simulink model "run_small_function_cov_bitadder"  (R2022b)
settings: Solver=VariableStepAuto  StartTime=0.0  StopTime=0.0  RelTol=1e-3
libraries: simulink x3193, hdlsllib x1590, ece1718_small_function x16
(part 4 of 26)

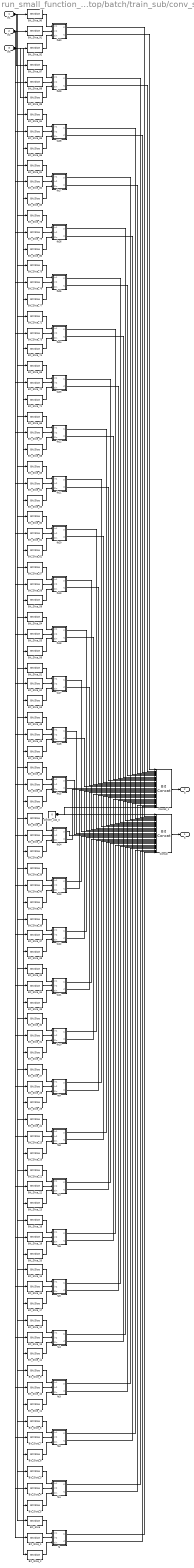
== system run_small_function_cov_bitadder/For Iterator Subsystem/train_top/batch/train_sub/conv_sig/filter dim iter /i ietar Subsystem/Subsystem/For Iterator Subsystem/mac/wt_multi/ca03 ==
  in1 : Inport  OutDataTypeStr=uint32  SampleTime=-1
  in2 : Inport  Port=2  OutDataTypeStr=uint32  SampleTime=-1
  in3 : Inport  Port=3  OutDataTypeStr=uint32  SampleTime=-1
  Bit_Slice : hdlsllib/Logic and Bit Operations/Bit Slice  lidx=double(0)  ridx=double(0)
  Bit_Slice_1 : hdlsllib/Logic and Bit Operations/Bit Slice  lidx=double(0)  ridx=double(0)
  Bit_Slice_10 : hdlsllib/Logic and Bit Operations/Bit Slice  lidx=double(3)  ridx=double(3)
  Bit_Slice_11 : hdlsllib/Logic and Bit Operations/Bit Slice  lidx=double(3)  ridx=double(3)
  Bit_Slice_12 : hdlsllib/Logic and Bit Operations/Bit Slice  lidx=double(4)  ridx=double(4)
  Bit_Slice_13 : hdlsllib/Logic and Bit Operations/Bit Slice  lidx=double(4)  ridx=double(4)
  Bit_Slice_14 : hdlsllib/Logic and Bit Operations/Bit Slice  lidx=double(4)  ridx=double(4)
  Bit_Slice_15 : hdlsllib/Logic and Bit Operations/Bit Slice  lidx=double(5)  ridx=double(5)
  Bit_Slice_16 : hdlsllib/Logic and Bit Operations/Bit Slice  lidx=double(5)  ridx=double(5)
  Bit_Slice_17 : hdlsllib/Logic and Bit Operations/Bit Slice  lidx=double(5)  ridx=double(5)
  Bit_Slice_18 : hdlsllib/Logic and Bit Operations/Bit Slice  lidx=double(6)  ridx=double(6)
  Bit_Slice_19 : hdlsllib/Logic and Bit Operations/Bit Slice  lidx=double(6)  ridx=double(6)
  Bit_Slice_2 : hdlsllib/Logic and Bit Operations/Bit Slice  lidx=double(0)  ridx=double(0)
  Bit_Slice_20 : hdlsllib/Logic and Bit Operations/Bit Slice  lidx=double(6)  ridx=double(6)
  Bit_Slice_21 : hdlsllib/Logic and Bit Operations/Bit Slice  lidx=double(7)  ridx=double(7)
  Bit_Slice_22 : hdlsllib/Logic and Bit Operations/Bit Slice  lidx=double(7)  ridx=double(7)
  Bit_Slice_23 : hdlsllib/Logic and Bit Operations/Bit Slice  lidx=double(7)  ridx=double(7)
  Bit_Slice_24 : hdlsllib/Logic and Bit Operations/Bit Slice  lidx=double(8)  ridx=double(8)
  Bit_Slice_25 : hdlsllib/Logic and Bit Operations/Bit Slice  lidx=double(8)  ridx=double(8)
  Bit_Slice_26 : hdlsllib/Logic and Bit Operations/Bit Slice  lidx=double(8)  ridx=double(8)
  Bit_Slice_27 : hdlsllib/Logic and Bit Operations/Bit Slice  lidx=double(9)  ridx=double(9)
  Bit_Slice_28 : hdlsllib/Logic and Bit Operations/Bit Slice  lidx=double(9)  ridx=double(9)
  Bit_Slice_29 : hdlsllib/Logic and Bit Operations/Bit Slice  lidx=double(9)  ridx=double(9)
  Bit_Slice_3 : hdlsllib/Logic and Bit Operations/Bit Slice  lidx=double(1)  ridx=double(1)
  Bit_Slice_30 : hdlsllib/Logic and Bit Operations/Bit Slice  lidx=double(10)  ridx=double(10)
  Bit_Slice_31 : hdlsllib/Logic and Bit Operations/Bit Slice  lidx=double(10)  ridx=double(10)
  Bit_Slice_32 : hdlsllib/Logic and Bit Operations/Bit Slice  lidx=double(10)  ridx=double(10)
  Bit_Slice_33 : hdlsllib/Logic and Bit Operations/Bit Slice  lidx=double(11)  ridx=double(11)
  Bit_Slice_34 : hdlsllib/Logic and Bit Operations/Bit Slice  lidx=double(11)  ridx=double(11)
  Bit_Slice_35 : hdlsllib/Logic and Bit Operations/Bit Slice  lidx=double(11)  ridx=double(11)
  Bit_Slice_36 : hdlsllib/Logic and Bit Operations/Bit Slice  lidx=double(12)  ridx=double(12)
  Bit_Slice_37 : hdlsllib/Logic and Bit Operations/Bit Slice  lidx=double(12)  ridx=double(12)
  Bit_Slice_38 : hdlsllib/Logic and Bit Operations/Bit Slice  lidx=double(12)  ridx=double(12)
  Bit_Slice_39 : hdlsllib/Logic and Bit Operations/Bit Slice  lidx=double(13)  ridx=double(13)
  Bit_Slice_4 : hdlsllib/Logic and Bit Operations/Bit Slice  lidx=double(1)  ridx=double(1)
  Bit_Slice_40 : hdlsllib/Logic and Bit Operations/Bit Slice  lidx=double(13)  ridx=double(13)
  Bit_Slice_41 : hdlsllib/Logic and Bit Operations/Bit Slice  lidx=double(13)  ridx=double(13)
  Bit_Slice_42 : hdlsllib/Logic and Bit Operations/Bit Slice  lidx=double(14)  ridx=double(14)
  Bit_Slice_43 : hdlsllib/Logic and Bit Operations/Bit Slice  lidx=double(14)  ridx=double(14)
  Bit_Slice_44 : hdlsllib/Logic and Bit Operations/Bit Slice  lidx=double(14)  ridx=double(14)
  Bit_Slice_45 : hdlsllib/Logic and Bit Operations/Bit Slice  lidx=double(15)  ridx=double(15)
  Bit_Slice_46 : hdlsllib/Logic and Bit Operations/Bit Slice  lidx=double(15)  ridx=double(15)
  Bit_Slice_47 : hdlsllib/Logic and Bit Operations/Bit Slice  lidx=double(15)  ridx=double(15)
  Bit_Slice_48 : hdlsllib/Logic and Bit Operations/Bit Slice  lidx=double(16)  ridx=double(16)
  Bit_Slice_49 : hdlsllib/Logic and Bit Operations/Bit Slice  lidx=double(16)  ridx=double(16)
  Bit_Slice_5 : hdlsllib/Logic and Bit Operations/Bit Slice  lidx=double(1)  ridx=double(1)
  Bit_Slice_50 : hdlsllib/Logic and Bit Operations/Bit Slice  lidx=double(16)  ridx=double(16)
  Bit_Slice_51 : hdlsllib/Logic and Bit Operations/Bit Slice  lidx=double(17)  ridx=double(17)
  Bit_Slice_52 : hdlsllib/Logic and Bit Operations/Bit Slice  lidx=double(17)  ridx=double(17)
  Bit_Slice_53 : hdlsllib/Logic and Bit Operations/Bit Slice  lidx=double(17)  ridx=double(17)
  Bit_Slice_54 : hdlsllib/Logic and Bit Operations/Bit Slice  lidx=double(18)  ridx=double(18)
  Bit_Slice_55 : hdlsllib/Logic and Bit Operations/Bit Slice  lidx=double(18)  ridx=double(18)
  Bit_Slice_56 : hdlsllib/Logic and Bit Operations/Bit Slice  lidx=double(18)  ridx=double(18)
  Bit_Slice_57 : hdlsllib/Logic and Bit Operations/Bit Slice  lidx=double(19)  ridx=double(19)
  Bit_Slice_58 : hdlsllib/Logic and Bit Operations/Bit Slice  lidx=double(19)  ridx=double(19)
  Bit_Slice_59 : hdlsllib/Logic and Bit Operations/Bit Slice  lidx=double(19)  ridx=double(19)
  Bit_Slice_6 : hdlsllib/Logic and Bit Operations/Bit Slice  lidx=double(2)  ridx=double(2)
  Bit_Slice_60 : hdlsllib/Logic and Bit Operations/Bit Slice  lidx=double(20)  ridx=double(20)
  Bit_Slice_61 : hdlsllib/Logic and Bit Operations/Bit Slice  lidx=double(20)  ridx=double(20)
  Bit_Slice_62 : hdlsllib/Logic and Bit Operations/Bit Slice  lidx=double(20)  ridx=double(20)
  Bit_Slice_63 : hdlsllib/Logic and Bit Operations/Bit Slice  lidx=double(21)  ridx=double(21)
  Bit_Slice_64 : hdlsllib/Logic and Bit Operations/Bit Slice  lidx=double(21)  ridx=double(21)
  Bit_Slice_65 : hdlsllib/Logic and Bit Operations/Bit Slice  lidx=double(21)  ridx=double(21)
  Bit_Slice_66 : hdlsllib/Logic and Bit Operations/Bit Slice  lidx=double(22)  ridx=double(22)
  Bit_Slice_67 : hdlsllib/Logic and Bit Operations/Bit Slice  lidx=double(22)  ridx=double(22)
  Bit_Slice_68 : hdlsllib/Logic and Bit Operations/Bit Slice  lidx=double(22)  ridx=double(22)
  Bit_Slice_69 : hdlsllib/Logic and Bit Operations/Bit Slice  lidx=double(23)  ridx=double(23)
  Bit_Slice_7 : hdlsllib/Logic and Bit Operations/Bit Slice  lidx=double(2)  ridx=double(2)
  Bit_Slice_70 : hdlsllib/Logic and Bit Operations/Bit Slice  lidx=double(23)  ridx=double(23)
  Bit_Slice_71 : hdlsllib/Logic and Bit Operations/Bit Slice  lidx=double(23)  ridx=double(23)
  Bit_Slice_72 : hdlsllib/Logic and Bit Operations/Bit Slice  lidx=double(24)  ridx=double(24)
  Bit_Slice_73 : hdlsllib/Logic and Bit Operations/Bit Slice  lidx=double(24)  ridx=double(24)
  Bit_Slice_74 : hdlsllib/Logic and Bit Operations/Bit Slice  lidx=double(24)  ridx=double(24)
  Bit_Slice_75 : hdlsllib/Logic and Bit Operations/Bit Slice  lidx=double(25)  ridx=double(25)
  Bit_Slice_76 : hdlsllib/Logic and Bit Operations/Bit Slice  lidx=double(25)  ridx=double(25)
  Bit_Slice_77 : hdlsllib/Logic and Bit Operations/Bit Slice  lidx=double(25)  ridx=double(25)
  Bit_Slice_78 : hdlsllib/Logic and Bit Operations/Bit Slice  lidx=double(26)  ridx=double(26)
  Bit_Slice_79 : hdlsllib/Logic and Bit Operations/Bit Slice  lidx=double(26)  ridx=double(26)
  Bit_Slice_8 : hdlsllib/Logic and Bit Operations/Bit Slice  lidx=double(2)  ridx=double(2)
  Bit_Slice_80 : hdlsllib/Logic and Bit Operations/Bit Slice  lidx=double(26)  ridx=double(26)
  Bit_Slice_81 : hdlsllib/Logic and Bit Operations/Bit Slice  lidx=double(27)  ridx=double(27)
  Bit_Slice_82 : hdlsllib/Logic and Bit Operations/Bit Slice  lidx=double(27)  ridx=double(27)
  Bit_Slice_83 : hdlsllib/Logic and Bit Operations/Bit Slice  lidx=double(27)  ridx=double(27)
  Bit_Slice_84 : hdlsllib/Logic and Bit Operations/Bit Slice  lidx=double(28)  ridx=double(28)
  Bit_Slice_85 : hdlsllib/Logic and Bit Operations/Bit Slice  lidx=double(28)  ridx=double(28)
  Bit_Slice_86 : hdlsllib/Logic and Bit Operations/Bit Slice  lidx=double(28)  ridx=double(28)
  Bit_Slice_87 : hdlsllib/Logic and Bit Operations/Bit Slice  lidx=double(29)  ridx=double(29)
  Bit_Slice_88 : hdlsllib/Logic and Bit Operations/Bit Slice  lidx=double(29)  ridx=double(29)
  Bit_Slice_89 : hdlsllib/Logic and Bit Operations/Bit Slice  lidx=double(29)  ridx=double(29)
  Bit_Slice_9 : hdlsllib/Logic and Bit Operations/Bit Slice  lidx=double(3)  ridx=double(3)
  Bit_Slice_90 : hdlsllib/Logic and Bit Operations/Bit Slice  lidx=double(30)  ridx=double(30)
  Bit_Slice_91 : hdlsllib/Logic and Bit Operations/Bit Slice  lidx=double(30)  ridx=double(30)
  Bit_Slice_92 : hdlsllib/Logic and Bit Operations/Bit Slice  lidx=double(30)  ridx=double(30)
  CONST_u1b_0 : Constant  Value=0  OutDataTypeStr=fixdt(0, 1, 0)  SampleTime=-1
  Concat : hdlsllib/Logic and Bit Operations/Bit Concat  numInputs=32
  Concat_1 : hdlsllib/Logic and Bit Operations/Bit Concat  numInputs=32
  fa : Subsystem
  fa1 : Subsystem
  fa10 : Subsystem
  fa11 : Subsystem
  fa12 : Subsystem
  fa13 : Subsystem
  fa14 : Subsystem
  fa15 : Subsystem
  fa16 : Subsystem
  fa17 : Subsystem
  fa18 : Subsystem
  fa19 : Subsystem
  fa2 : Subsystem
  fa20 : Subsystem
  fa21 : Subsystem
  fa22 : Subsystem
  fa23 : Subsystem
  fa24 : Subsystem
  fa25 : Subsystem
  fa26 : Subsystem
  fa27 : Subsystem
  fa28 : Subsystem
  fa29 : Subsystem
  fa3 : Subsystem
  fa30 : Subsystem
  fa4 : Subsystem
  fa5 : Subsystem
  fa6 : Subsystem
  fa7 : Subsystem
  fa8 : Subsystem
  fa9 : Subsystem
  S : Outport  OutDataTypeStr=uint32  SampleTime=-1
  C : Outport  Port=2  OutDataTypeStr=uint32  SampleTime=-1
  wires:
  in2/1 -> Bit_Slice_91/1, Bit_Slice_88/1, Bit_Slice_85/1, Bit_Slice_82/1, Bit_Slice_79/1, Bit_Slice_76/1, Bit_Slice_73/1, Bit_Slice_70/1, Bit_Slice_67/1, Bit_Slice_64/1, Bit_Slice_61/1, Bit_Slice_58/1, Bit_Slice_55/1, Bit_Slice_52/1, Bit_Slice_49/1, Bit_Slice_46/1, Bit_Slice_43/1, Bit_Slice_40/1, Bit_Slice_37/1, Bit_Slice_34/1, Bit_Slice_31/1, Bit_Slice_28/1, Bit_Slice_25/1, Bit_Slice_22/1, Bit_Slice_19/1, Bit_Slice_16/1, Bit_Slice_13/1, Bit_Slice_10/1, Bit_Slice_7/1, Bit_Slice_4/1, Bit_Slice_1/1
  Concat_1/1 -> C/1
  Bit_Slice_2/1 -> fa/3(Cin)
  fa/1(S) -> Concat/32
  fa1/2(C) -> Concat_1/30
  Bit_Slice_8/1 -> fa2/3(Cin)
  fa2/2(C) -> Concat_1/29
  Bit_Slice_9/1 -> fa3/1(in1)
  Bit_Slice_10/1 -> fa3/2(in2)
  Bit_Slice_11/1 -> fa3/3(Cin)
  fa4/2(C) -> Concat_1/27
  Bit_Slice_16/1 -> fa5/2(in2)
  Bit_Slice_17/1 -> fa5/3(Cin)
  fa5/2(C) -> Concat_1/26
  Bit_Slice_18/1 -> fa6/1(in1)
  fa6/1(S) -> Concat/26
  fa7/1(S) -> Concat/25
  Bit_Slice_24/1 -> fa8/1(in1)
  fa8/2(C) -> Concat_1/23
  Bit_Slice_27/1 -> fa9/1(in1)
  Bit_Slice_28/1 -> fa9/2(in2)
  Bit_Slice_30/1 -> fa10/1(in1)
  Bit_Slice_32/1 -> fa10/3(Cin)
  Bit_Slice_4/1 -> fa1/2(in2)
  fa10/1(S) -> Concat/22
  Bit_Slice_33/1 -> fa11/1(in1)
  Bit_Slice_34/1 -> fa11/2(in2)
  Bit_Slice_35/1 -> fa11/3(Cin)
  fa11/1(S) -> Concat/21
  fa11/2(C) -> Concat_1/20
  fa6/2(C) -> Concat_1/25
  Bit_Slice_38/1 -> fa12/3(Cin)
  in3/1 -> Bit_Slice_92/1, Bit_Slice_89/1, Bit_Slice_86/1, Bit_Slice_83/1, Bit_Slice_80/1, Bit_Slice_77/1, Bit_Slice_74/1, Bit_Slice_71/1, Bit_Slice_68/1, Bit_Slice_65/1, Bit_Slice_62/1, Bit_Slice_59/1, Bit_Slice_56/1, Bit_Slice_53/1, Bit_Slice_50/1, Bit_Slice_47/1, Bit_Slice_44/1, Bit_Slice_41/1, Bit_Slice_38/1, Bit_Slice_35/1, Bit_Slice_32/1, Bit_Slice_29/1, Bit_Slice_26/1, Bit_Slice_23/1, Bit_Slice_20/1, Bit_Slice_17/1, Bit_Slice_14/1, Bit_Slice_11/1, Bit_Slice_8/1, Bit_Slice_5/1, Bit_Slice_2/1
  Bit_Slice_23/1 -> fa7/3(Cin)
  fa12/1(S) -> Concat/20
  fa12/2(C) -> Concat_1/19
  fa5/1(S) -> Concat/27
  Bit_Slice_39/1 -> fa13/1(in1)
  Bit_Slice_41/1 -> fa13/3(Cin)
  fa13/2(C) -> Concat_1/18
  Bit_Slice_43/1 -> fa14/2(in2)
  Bit_Slice_44/1 -> fa14/3(Cin)
  fa/2(C) -> Concat_1/31
  fa14/1(S) -> Concat/18
  Bit_Slice_45/1 -> fa15/1(in1)
  Bit_Slice_40/1 -> fa13/2(in2)
  Bit_Slice_46/1 -> fa15/2(in2)
  Bit_Slice_85/1 -> fa28/2(in2)
  fa9/2(C) -> Concat_1/22
  Bit_Slice_48/1 -> fa16/1(in1)
  Bit_Slice_5/1 -> fa1/3(Cin)
  Bit_Slice_15/1 -> fa5/1(in1)
  fa24/2(C) -> Concat_1/7
  fa4/1(S) -> Concat/28
  Bit_Slice_72/1 -> fa24/1(in1)
  Bit_Slice_71/1 -> fa23/3(Cin)
  Bit_Slice_77/1 -> fa25/3(Cin)
  Bit_Slice_90/1 -> fa30/1(in1)
  fa1/1(S) -> Concat/31
  Bit_Slice_69/1 -> fa23/1(in1)
  Bit_Slice_59/1 -> fa19/3(Cin)
  CONST_u1b_0/1 -> Concat_1/32, Concat/1
  fa28/1(S) -> Concat/4
  fa25/2(C) -> Concat_1/6
  Bit_Slice_29/1 -> fa9/3(Cin)
  Bit_Slice_78/1 -> fa26/1(in1)
  Concat/1 -> S/1
  Bit_Slice_42/1 -> fa14/1(in1)
  Bit_Slice_70/1 -> fa23/2(in2)
  fa24/1(S) -> Concat/8
  fa26/2(C) -> Concat_1/5
  Bit_Slice_58/1 -> fa19/2(in2)
  Bit_Slice_82/1 -> fa27/2(in2)
  in1/1 -> Bit_Slice_90/1, Bit_Slice_87/1, Bit_Slice_84/1, Bit_Slice_81/1, Bit_Slice_78/1, Bit_Slice_75/1, Bit_Slice_72/1, Bit_Slice_69/1, Bit_Slice_66/1, Bit_Slice_63/1, Bit_Slice_60/1, Bit_Slice_57/1, Bit_Slice_54/1, Bit_Slice_51/1, Bit_Slice_48/1, Bit_Slice_45/1, Bit_Slice_42/1, Bit_Slice_39/1, Bit_Slice_36/1, Bit_Slice_33/1, Bit_Slice_30/1, Bit_Slice_27/1, Bit_Slice_24/1, Bit_Slice_21/1, Bit_Slice_18/1, Bit_Slice_15/1, Bit_Slice_12/1, Bit_Slice_9/1, Bit_Slice_6/1, Bit_Slice_3/1, Bit_Slice/1
  Bit_Slice_87/1 -> fa29/1(in1)
  fa27/1(S) -> Concat/5
  Bit_Slice_55/1 -> fa18/2(in2)
  fa21/2(C) -> Concat_1/10
  Bit_Slice_79/1 -> fa26/2(in2)
  Bit_Slice_92/1 -> fa30/3(Cin)
  fa2/1(S) -> Concat/30
  Bit_Slice_56/1 -> fa18/3(Cin)
  Bit_Slice_80/1 -> fa26/3(Cin)
  fa20/1(S) -> Concat/12
  Bit_Slice_53/1 -> fa17/3(Cin)
  Bit_Slice_26/1 -> fa8/3(Cin)
  Bit_Slice_51/1 -> fa17/1(in1)
  Bit_Slice_25/1 -> fa8/2(in2)
  fa30/2(C) -> Concat_1/1
  Bit_Slice_73/1 -> fa24/2(in2)
  fa30/1(S) -> Concat/2
  Bit_Slice/1 -> fa/1(in1)
  Bit_Slice_37/1 -> fa12/2(in2)
  fa16/1(S) -> Concat/16
  fa25/1(S) -> Concat/7
  fa26/1(S) -> Concat/6
  Bit_Slice_86/1 -> fa28/3(Cin)
  Bit_Slice_74/1 -> fa24/3(Cin)
  Bit_Slice_14/1 -> fa4/3(Cin)
  fa29/2(C) -> Concat_1/2
  Bit_Slice_83/1 -> fa27/3(Cin)
  fa20/2(C) -> Concat_1/11
  fa19/1(S) -> Concat/13
  Bit_Slice_31/1 -> fa10/2(in2)
  Bit_Slice_88/1 -> fa29/2(in2)
  fa8/1(S) -> Concat/24
  Bit_Slice_76/1 -> fa25/2(in2)
  Bit_Slice_81/1 -> fa27/1(in1)
  fa29/1(S) -> Concat/3
  Bit_Slice_7/1 -> fa2/2(in2)
  fa18/1(S) -> Concat/14
  fa28/2(C) -> Concat_1/3
  fa23/1(S) -> Concat/9
  fa14/2(C) -> Concat_1/17
  Bit_Slice_66/1 -> fa22/1(in1)
  fa22/1(S) -> Concat/10
  Bit_Slice_64/1 -> fa21/2(in2)
  Bit_Slice_6/1 -> fa2/1(in1)
  Bit_Slice_19/1 -> fa6/2(in2)
  fa9/1(S) -> Concat/23
  Bit_Slice_52/1 -> fa17/2(in2)
  Bit_Slice_89/1 -> fa29/3(Cin)
  fa22/2(C) -> Concat_1/9
  Bit_Slice_91/1 -> fa30/2(in2)
  Bit_Slice_68/1 -> fa22/3(Cin)
  Bit_Slice_67/1 -> fa22/2(in2)
  fa3/2(C) -> Concat_1/28
  fa21/1(S) -> Concat/11
  Bit_Slice_36/1 -> fa12/1(in1)
  fa27/2(C) -> Concat_1/4
  Bit_Slice_61/1 -> fa20/2(in2)
  Bit_Slice_50/1 -> fa16/3(Cin)
  Bit_Slice_63/1 -> fa21/1(in1)
  Bit_Slice_1/1 -> fa/2(in2)
  Bit_Slice_60/1 -> fa20/1(in1)
  Bit_Slice_21/1 -> fa7/1(in1)
  Bit_Slice_84/1 -> fa28/1(in1)
  fa19/2(C) -> Concat_1/12
  Bit_Slice_12/1 -> fa4/1(in1)
  Bit_Slice_20/1 -> fa6/3(Cin)
  Bit_Slice_57/1 -> fa19/1(in1)
  Bit_Slice_22/1 -> fa7/2(in2)
  fa7/2(C) -> Concat_1/24
  Bit_Slice_54/1 -> fa18/1(in1)
  fa23/2(C) -> Concat_1/8
  fa18/2(C) -> Concat_1/13
  fa15/2(C) -> Concat_1/16
  fa17/2(C) -> Concat_1/14
  fa10/2(C) -> Concat_1/21
  fa13/1(S) -> Concat/19
  fa17/1(S) -> Concat/15
  fa16/2(C) -> Concat_1/15
  fa3/1(S) -> Concat/29
  Bit_Slice_75/1 -> fa25/1(in1)
  Bit_Slice_65/1 -> fa21/3(Cin)
  Bit_Slice_49/1 -> fa16/2(in2)
  Bit_Slice_3/1 -> fa1/1(in1)
  fa15/1(S) -> Concat/17
  Bit_Slice_13/1 -> fa4/2(in2)
  Bit_Slice_62/1 -> fa20/3(Cin)
  Bit_Slice_47/1 -> fa15/3(Cin)

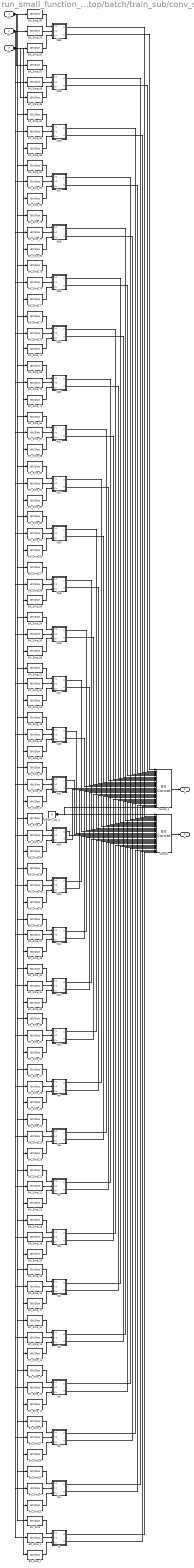
== system run_small_function_cov_bitadder/For Iterator Subsystem/train_top/batch/train_sub/conv_sig/filter dim iter /i ietar Subsystem/Subsystem/For Iterator Subsystem/mac/wt_multi/ca04 ==
  in1 : Inport  OutDataTypeStr=uint32  SampleTime=-1
  in2 : Inport  Port=2  OutDataTypeStr=uint32  SampleTime=-1
  in3 : Inport  Port=3  OutDataTypeStr=uint32  SampleTime=-1
  Bit_Slice : hdlsllib/Logic and Bit Operations/Bit Slice  lidx=double(0)  ridx=double(0)
  Bit_Slice_1 : hdlsllib/Logic and Bit Operations/Bit Slice  lidx=double(0)  ridx=double(0)
  Bit_Slice_10 : hdlsllib/Logic and Bit Operations/Bit Slice  lidx=double(3)  ridx=double(3)
  Bit_Slice_11 : hdlsllib/Logic and Bit Operations/Bit Slice  lidx=double(3)  ridx=double(3)
  Bit_Slice_12 : hdlsllib/Logic and Bit Operations/Bit Slice  lidx=double(4)  ridx=double(4)
  Bit_Slice_13 : hdlsllib/Logic and Bit Operations/Bit Slice  lidx=double(4)  ridx=double(4)
  Bit_Slice_14 : hdlsllib/Logic and Bit Operations/Bit Slice  lidx=double(4)  ridx=double(4)
  Bit_Slice_15 : hdlsllib/Logic and Bit Operations/Bit Slice  lidx=double(5)  ridx=double(5)
  Bit_Slice_16 : hdlsllib/Logic and Bit Operations/Bit Slice  lidx=double(5)  ridx=double(5)
  Bit_Slice_17 : hdlsllib/Logic and Bit Operations/Bit Slice  lidx=double(5)  ridx=double(5)
  Bit_Slice_18 : hdlsllib/Logic and Bit Operations/Bit Slice  lidx=double(6)  ridx=double(6)
  Bit_Slice_19 : hdlsllib/Logic and Bit Operations/Bit Slice  lidx=double(6)  ridx=double(6)
  Bit_Slice_2 : hdlsllib/Logic and Bit Operations/Bit Slice  lidx=double(0)  ridx=double(0)
  Bit_Slice_20 : hdlsllib/Logic and Bit Operations/Bit Slice  lidx=double(6)  ridx=double(6)
  Bit_Slice_21 : hdlsllib/Logic and Bit Operations/Bit Slice  lidx=double(7)  ridx=double(7)
  Bit_Slice_22 : hdlsllib/Logic and Bit Operations/Bit Slice  lidx=double(7)  ridx=double(7)
  Bit_Slice_23 : hdlsllib/Logic and Bit Operations/Bit Slice  lidx=double(7)  ridx=double(7)
  Bit_Slice_24 : hdlsllib/Logic and Bit Operations/Bit Slice  lidx=double(8)  ridx=double(8)
  Bit_Slice_25 : hdlsllib/Logic and Bit Operations/Bit Slice  lidx=double(8)  ridx=double(8)
  Bit_Slice_26 : hdlsllib/Logic and Bit Operations/Bit Slice  lidx=double(8)  ridx=double(8)
  Bit_Slice_27 : hdlsllib/Logic and Bit Operations/Bit Slice  lidx=double(9)  ridx=double(9)
  Bit_Slice_28 : hdlsllib/Logic and Bit Operations/Bit Slice  lidx=double(9)  ridx=double(9)
  Bit_Slice_29 : hdlsllib/Logic and Bit Operations/Bit Slice  lidx=double(9)  ridx=double(9)
  Bit_Slice_3 : hdlsllib/Logic and Bit Operations/Bit Slice  lidx=double(1)  ridx=double(1)
  Bit_Slice_30 : hdlsllib/Logic and Bit Operations/Bit Slice  lidx=double(10)  ridx=double(10)
  Bit_Slice_31 : hdlsllib/Logic and Bit Operations/Bit Slice  lidx=double(10)  ridx=double(10)
  Bit_Slice_32 : hdlsllib/Logic and Bit Operations/Bit Slice  lidx=double(10)  ridx=double(10)
  Bit_Slice_33 : hdlsllib/Logic and Bit Operations/Bit Slice  lidx=double(11)  ridx=double(11)
  Bit_Slice_34 : hdlsllib/Logic and Bit Operations/Bit Slice  lidx=double(11)  ridx=double(11)
  Bit_Slice_35 : hdlsllib/Logic and Bit Operations/Bit Slice  lidx=double(11)  ridx=double(11)
  Bit_Slice_36 : hdlsllib/Logic and Bit Operations/Bit Slice  lidx=double(12)  ridx=double(12)
  Bit_Slice_37 : hdlsllib/Logic and Bit Operations/Bit Slice  lidx=double(12)  ridx=double(12)
  Bit_Slice_38 : hdlsllib/Logic and Bit Operations/Bit Slice  lidx=double(12)  ridx=double(12)
  Bit_Slice_39 : hdlsllib/Logic and Bit Operations/Bit Slice  lidx=double(13)  ridx=double(13)
  Bit_Slice_4 : hdlsllib/Logic and Bit Operations/Bit Slice  lidx=double(1)  ridx=double(1)
  Bit_Slice_40 : hdlsllib/Logic and Bit Operations/Bit Slice  lidx=double(13)  ridx=double(13)
  Bit_Slice_41 : hdlsllib/Logic and Bit Operations/Bit Slice  lidx=double(13)  ridx=double(13)
  Bit_Slice_42 : hdlsllib/Logic and Bit Operations/Bit Slice  lidx=double(14)  ridx=double(14)
  Bit_Slice_43 : hdlsllib/Logic and Bit Operations/Bit Slice  lidx=double(14)  ridx=double(14)
  Bit_Slice_44 : hdlsllib/Logic and Bit Operations/Bit Slice  lidx=double(14)  ridx=double(14)
  Bit_Slice_45 : hdlsllib/Logic and Bit Operations/Bit Slice  lidx=double(15)  ridx=double(15)
  Bit_Slice_46 : hdlsllib/Logic and Bit Operations/Bit Slice  lidx=double(15)  ridx=double(15)
  Bit_Slice_47 : hdlsllib/Logic and Bit Operations/Bit Slice  lidx=double(15)  ridx=double(15)
  Bit_Slice_48 : hdlsllib/Logic and Bit Operations/Bit Slice  lidx=double(16)  ridx=double(16)
  Bit_Slice_49 : hdlsllib/Logic and Bit Operations/Bit Slice  lidx=double(16)  ridx=double(16)
  Bit_Slice_5 : hdlsllib/Logic and Bit Operations/Bit Slice  lidx=double(1)  ridx=double(1)
  Bit_Slice_50 : hdlsllib/Logic and Bit Operations/Bit Slice  lidx=double(16)  ridx=double(16)
  Bit_Slice_51 : hdlsllib/Logic and Bit Operations/Bit Slice  lidx=double(17)  ridx=double(17)
  Bit_Slice_52 : hdlsllib/Logic and Bit Operations/Bit Slice  lidx=double(17)  ridx=double(17)
  Bit_Slice_53 : hdlsllib/Logic and Bit Operations/Bit Slice  lidx=double(17)  ridx=double(17)
  Bit_Slice_54 : hdlsllib/Logic and Bit Operations/Bit Slice  lidx=double(18)  ridx=double(18)
  Bit_Slice_55 : hdlsllib/Logic and Bit Operations/Bit Slice  lidx=double(18)  ridx=double(18)
  Bit_Slice_56 : hdlsllib/Logic and Bit Operations/Bit Slice  lidx=double(18)  ridx=double(18)
  Bit_Slice_57 : hdlsllib/Logic and Bit Operations/Bit Slice  lidx=double(19)  ridx=double(19)
  Bit_Slice_58 : hdlsllib/Logic and Bit Operations/Bit Slice  lidx=double(19)  ridx=double(19)
  Bit_Slice_59 : hdlsllib/Logic and Bit Operations/Bit Slice  lidx=double(19)  ridx=double(19)
  Bit_Slice_6 : hdlsllib/Logic and Bit Operations/Bit Slice  lidx=double(2)  ridx=double(2)
  Bit_Slice_60 : hdlsllib/Logic and Bit Operations/Bit Slice  lidx=double(20)  ridx=double(20)
  Bit_Slice_61 : hdlsllib/Logic and Bit Operations/Bit Slice  lidx=double(20)  ridx=double(20)
  Bit_Slice_62 : hdlsllib/Logic and Bit Operations/Bit Slice  lidx=double(20)  ridx=double(20)
  Bit_Slice_63 : hdlsllib/Logic and Bit Operations/Bit Slice  lidx=double(21)  ridx=double(21)
  Bit_Slice_64 : hdlsllib/Logic and Bit Operations/Bit Slice  lidx=double(21)  ridx=double(21)
  Bit_Slice_65 : hdlsllib/Logic and Bit Operations/Bit Slice  lidx=double(21)  ridx=double(21)
  Bit_Slice_66 : hdlsllib/Logic and Bit Operations/Bit Slice  lidx=double(22)  ridx=double(22)
  Bit_Slice_67 : hdlsllib/Logic and Bit Operations/Bit Slice  lidx=double(22)  ridx=double(22)
  Bit_Slice_68 : hdlsllib/Logic and Bit Operations/Bit Slice  lidx=double(22)  ridx=double(22)
  Bit_Slice_69 : hdlsllib/Logic and Bit Operations/Bit Slice  lidx=double(23)  ridx=double(23)
  Bit_Slice_7 : hdlsllib/Logic and Bit Operations/Bit Slice  lidx=double(2)  ridx=double(2)
  Bit_Slice_70 : hdlsllib/Logic and Bit Operations/Bit Slice  lidx=double(23)  ridx=double(23)
  Bit_Slice_71 : hdlsllib/Logic and Bit Operations/Bit Slice  lidx=double(23)  ridx=double(23)
  Bit_Slice_72 : hdlsllib/Logic and Bit Operations/Bit Slice  lidx=double(24)  ridx=double(24)
  Bit_Slice_73 : hdlsllib/Logic and Bit Operations/Bit Slice  lidx=double(24)  ridx=double(24)
  Bit_Slice_74 : hdlsllib/Logic and Bit Operations/Bit Slice  lidx=double(24)  ridx=double(24)
  Bit_Slice_75 : hdlsllib/Logic and Bit Operations/Bit Slice  lidx=double(25)  ridx=double(25)
  Bit_Slice_76 : hdlsllib/Logic and Bit Operations/Bit Slice  lidx=double(25)  ridx=double(25)
  Bit_Slice_77 : hdlsllib/Logic and Bit Operations/Bit Slice  lidx=double(25)  ridx=double(25)
  Bit_Slice_78 : hdlsllib/Logic and Bit Operations/Bit Slice  lidx=double(26)  ridx=double(26)
  Bit_Slice_79 : hdlsllib/Logic and Bit Operations/Bit Slice  lidx=double(26)  ridx=double(26)
  Bit_Slice_8 : hdlsllib/Logic and Bit Operations/Bit Slice  lidx=double(2)  ridx=double(2)
  Bit_Slice_80 : hdlsllib/Logic and Bit Operations/Bit Slice  lidx=double(26)  ridx=double(26)
  Bit_Slice_81 : hdlsllib/Logic and Bit Operations/Bit Slice  lidx=double(27)  ridx=double(27)
  Bit_Slice_82 : hdlsllib/Logic and Bit Operations/Bit Slice  lidx=double(27)  ridx=double(27)
  Bit_Slice_83 : hdlsllib/Logic and Bit Operations/Bit Slice  lidx=double(27)  ridx=double(27)
  Bit_Slice_84 : hdlsllib/Logic and Bit Operations/Bit Slice  lidx=double(28)  ridx=double(28)
  Bit_Slice_85 : hdlsllib/Logic and Bit Operations/Bit Slice  lidx=double(28)  ridx=double(28)
  Bit_Slice_86 : hdlsllib/Logic and Bit Operations/Bit Slice  lidx=double(28)  ridx=double(28)
  Bit_Slice_87 : hdlsllib/Logic and Bit Operations/Bit Slice  lidx=double(29)  ridx=double(29)
  Bit_Slice_88 : hdlsllib/Logic and Bit Operations/Bit Slice  lidx=double(29)  ridx=double(29)
  Bit_Slice_89 : hdlsllib/Logic and Bit Operations/Bit Slice  lidx=double(29)  ridx=double(29)
  Bit_Slice_9 : hdlsllib/Logic and Bit Operations/Bit Slice  lidx=double(3)  ridx=double(3)
  Bit_Slice_90 : hdlsllib/Logic and Bit Operations/Bit Slice  lidx=double(30)  ridx=double(30)
  Bit_Slice_91 : hdlsllib/Logic and Bit Operations/Bit Slice  lidx=double(30)  ridx=double(30)
  Bit_Slice_92 : hdlsllib/Logic and Bit Operations/Bit Slice  lidx=double(30)  ridx=double(30)
  CONST_u1b_0 : Constant  Value=0  OutDataTypeStr=fixdt(0, 1, 0)  SampleTime=-1
  Concat : hdlsllib/Logic and Bit Operations/Bit Concat  numInputs=32
  Concat_1 : hdlsllib/Logic and Bit Operations/Bit Concat  numInputs=32
  fa : Subsystem
  fa1 : Subsystem
  fa10 : Subsystem
  fa11 : Subsystem
  fa12 : Subsystem
  fa13 : Subsystem
  fa14 : Subsystem
  fa15 : Subsystem
  fa16 : Subsystem
  fa17 : Subsystem
  fa18 : Subsystem
  fa19 : Subsystem
  fa2 : Subsystem
  fa20 : Subsystem
  fa21 : Subsystem
  fa22 : Subsystem
  fa23 : Subsystem
  fa24 : Subsystem
  fa25 : Subsystem
  fa26 : Subsystem
  fa27 : Subsystem
  fa28 : Subsystem
  fa29 : Subsystem
  fa3 : Subsystem
  fa30 : Subsystem
  fa4 : Subsystem
  fa5 : Subsystem
  fa6 : Subsystem
  fa7 : Subsystem
  fa8 : Subsystem
  fa9 : Subsystem
  S : Outport  OutDataTypeStr=uint32  SampleTime=-1
  C : Outport  Port=2  OutDataTypeStr=uint32  SampleTime=-1
  wires:
  in1/1 -> Bit_Slice_90/1, Bit_Slice_87/1, Bit_Slice_84/1, Bit_Slice_81/1, Bit_Slice_78/1, Bit_Slice_75/1, Bit_Slice_72/1, Bit_Slice_69/1, Bit_Slice_66/1, Bit_Slice_63/1, Bit_Slice_60/1, Bit_Slice_57/1, Bit_Slice_54/1, Bit_Slice_51/1, Bit_Slice_48/1, Bit_Slice_45/1, Bit_Slice_42/1, Bit_Slice_39/1, Bit_Slice_36/1, Bit_Slice_33/1, Bit_Slice_30/1, Bit_Slice_27/1, Bit_Slice_24/1, Bit_Slice_21/1, Bit_Slice_18/1, Bit_Slice_15/1, Bit_Slice_12/1, Bit_Slice_9/1, Bit_Slice_6/1, Bit_Slice_3/1, Bit_Slice/1
  in2/1 -> Bit_Slice_91/1, Bit_Slice_88/1, Bit_Slice_85/1, Bit_Slice_82/1, Bit_Slice_79/1, Bit_Slice_76/1, Bit_Slice_73/1, Bit_Slice_70/1, Bit_Slice_67/1, Bit_Slice_64/1, Bit_Slice_61/1, Bit_Slice_58/1, Bit_Slice_55/1, Bit_Slice_52/1, Bit_Slice_49/1, Bit_Slice_46/1, Bit_Slice_43/1, Bit_Slice_40/1, Bit_Slice_37/1, Bit_Slice_34/1, Bit_Slice_31/1, Bit_Slice_28/1, Bit_Slice_25/1, Bit_Slice_22/1, Bit_Slice_19/1, Bit_Slice_16/1, Bit_Slice_13/1, Bit_Slice_10/1, Bit_Slice_7/1, Bit_Slice_4/1, Bit_Slice_1/1
  Concat/1 -> S/1
  Bit_Slice/1 -> fa/1(in1)
  Bit_Slice_2/1 -> fa/3(Cin)
  fa/1(S) -> Concat/32
  Bit_Slice_3/1 -> fa1/1(in1)
  fa1/2(C) -> Concat_1/30
  Bit_Slice_7/1 -> fa2/2(in2)
  Bit_Slice_9/1 -> fa3/1(in1)
  Bit_Slice_10/1 -> fa3/2(in2)
  Bit_Slice_11/1 -> fa3/3(Cin)
  fa3/1(S) -> Concat/29
  Bit_Slice_14/1 -> fa4/3(Cin)
  fa/2(C) -> Concat_1/31
  Bit_Slice_16/1 -> fa5/2(in2)
  fa4/1(S) -> Concat/28
  Bit_Slice_17/1 -> fa5/3(Cin)
  Bit_Slice_12/1 -> fa4/1(in1)
  fa5/1(S) -> Concat/27
  fa5/2(C) -> Concat_1/26
  Bit_Slice_20/1 -> fa6/3(Cin)
  Bit_Slice_22/1 -> fa7/2(in2)
  Bit_Slice_23/1 -> fa7/3(Cin)
  Bit_Slice_1/1 -> fa/2(in2)
  fa7/1(S) -> Concat/25
  fa7/2(C) -> Concat_1/24
  Bit_Slice_25/1 -> fa8/2(in2)
  Bit_Slice_27/1 -> fa9/1(in1)
  Bit_Slice_28/1 -> fa9/2(in2)
  fa9/2(C) -> Concat_1/22
  Bit_Slice_19/1 -> fa6/2(in2)
  Bit_Slice_31/1 -> fa10/2(in2)
  Concat_1/1 -> C/1
  Bit_Slice_32/1 -> fa10/3(Cin)
  Bit_Slice_13/1 -> fa4/2(in2)
  fa10/1(S) -> Concat/22
  fa11/2(C) -> Concat_1/20
  Bit_Slice_21/1 -> fa7/1(in1)
  Bit_Slice_37/1 -> fa12/2(in2)
  Bit_Slice_38/1 -> fa12/3(Cin)
  fa12/2(C) -> Concat_1/19
  Bit_Slice_39/1 -> fa13/1(in1)
  Bit_Slice_40/1 -> fa13/2(in2)
  Bit_Slice_41/1 -> fa13/3(Cin)
  fa13/2(C) -> Concat_1/18
  Bit_Slice_18/1 -> fa6/1(in1)
  fa10/2(C) -> Concat_1/21
  fa14/1(S) -> Concat/18
  fa14/2(C) -> Concat_1/17
  Bit_Slice_45/1 -> fa15/1(in1)
  Bit_Slice_46/1 -> fa15/2(in2)
  fa2/2(C) -> Concat_1/29
  fa26/2(C) -> Concat_1/5
  fa16/2(C) -> Concat_1/15
  Bit_Slice_74/1 -> fa24/3(Cin)
  fa24/2(C) -> Concat_1/7
  Bit_Slice_75/1 -> fa25/1(in1)
  Bit_Slice_73/1 -> fa24/2(in2)
  fa25/1(S) -> Concat/7
  fa8/2(C) -> Concat_1/23
  Bit_Slice_42/1 -> fa14/1(in1)
  Bit_Slice_57/1 -> fa19/1(in1)
  Bit_Slice_79/1 -> fa26/2(in2)
  fa6/2(C) -> Concat_1/25
  fa19/1(S) -> Concat/13
  Bit_Slice_80/1 -> fa26/3(Cin)
  fa26/1(S) -> Concat/6
  fa18/1(S) -> Concat/14
  Bit_Slice_34/1 -> fa11/2(in2)
  Bit_Slice_82/1 -> fa27/2(in2)
  fa17/1(S) -> Concat/15
  Bit_Slice_44/1 -> fa14/3(Cin)
  Bit_Slice_90/1 -> fa30/1(in1)
  fa29/2(C) -> Concat_1/2
  Bit_Slice_15/1 -> fa5/1(in1)
  fa30/2(C) -> Concat_1/1
  Bit_Slice_77/1 -> fa25/3(Cin)
  fa29/1(S) -> Concat/3
  fa12/1(S) -> Concat/20
  Bit_Slice_58/1 -> fa19/2(in2)
  Bit_Slice_78/1 -> fa26/1(in1)
  Bit_Slice_72/1 -> fa24/1(in1)
  Bit_Slice_88/1 -> fa29/2(in2)
  Bit_Slice_5/1 -> fa1/3(Cin)
  Bit_Slice_91/1 -> fa30/2(in2)
  fa25/2(C) -> Concat_1/6
  fa19/2(C) -> Concat_1/12
  Bit_Slice_26/1 -> fa8/3(Cin)
  Bit_Slice_87/1 -> fa29/1(in1)
  Bit_Slice_6/1 -> fa2/1(in1)
  Bit_Slice_64/1 -> fa21/2(in2)
  fa13/1(S) -> Concat/19
  fa24/1(S) -> Concat/8
  fa20/1(S) -> Concat/12
  Bit_Slice_29/1 -> fa9/3(Cin)
  Bit_Slice_85/1 -> fa28/2(in2)
  fa9/1(S) -> Concat/23
  Bit_Slice_63/1 -> fa21/1(in1)
  Bit_Slice_84/1 -> fa28/1(in1)
  fa28/2(C) -> Concat_1/3
  Bit_Slice_86/1 -> fa28/3(Cin)
  fa27/2(C) -> Concat_1/4
  Bit_Slice_49/1 -> fa16/2(in2)
  Bit_Slice_48/1 -> fa16/1(in1)
  fa28/1(S) -> Concat/4
  Bit_Slice_71/1 -> fa23/3(Cin)
  Bit_Slice_76/1 -> fa25/2(in2)
  Bit_Slice_70/1 -> fa23/2(in2)
  Bit_Slice_89/1 -> fa29/3(Cin)
  fa16/1(S) -> Concat/16
  Bit_Slice_43/1 -> fa14/2(in2)
  Bit_Slice_83/1 -> fa27/3(Cin)
  fa23/1(S) -> Concat/9
  Bit_Slice_69/1 -> fa23/1(in1)
  Bit_Slice_61/1 -> fa20/2(in2)
  fa18/2(C) -> Concat_1/13
  fa15/1(S) -> Concat/17
  fa22/1(S) -> Concat/10
  Bit_Slice_8/1 -> fa2/3(Cin)
  Bit_Slice_68/1 -> fa22/3(Cin)
  fa21/2(C) -> Concat_1/10
  Bit_Slice_67/1 -> fa22/2(in2)
  Bit_Slice_4/1 -> fa1/2(in2)
  Bit_Slice_66/1 -> fa22/1(in1)
  fa1/1(S) -> Concat/31
  fa21/1(S) -> Concat/11
  fa20/2(C) -> Concat_1/11
  fa2/1(S) -> Concat/30
  fa4/2(C) -> Concat_1/27
  fa30/1(S) -> Concat/2
  Bit_Slice_65/1 -> fa21/3(Cin)
  Bit_Slice_24/1 -> fa8/1(in1)
  Bit_Slice_36/1 -> fa12/1(in1)
  Bit_Slice_60/1 -> fa20/1(in1)
  fa23/2(C) -> Concat_1/8
  Bit_Slice_62/1 -> fa20/3(Cin)
  fa6/1(S) -> Concat/26
  Bit_Slice_59/1 -> fa19/3(Cin)
  Bit_Slice_56/1 -> fa18/3(Cin)
  Bit_Slice_92/1 -> fa30/3(Cin)
  Bit_Slice_81/1 -> fa27/1(in1)
  Bit_Slice_55/1 -> fa18/2(in2)
  Bit_Slice_33/1 -> fa11/1(in1)
  Bit_Slice_54/1 -> fa18/1(in1)
  fa27/1(S) -> Concat/5
  fa22/2(C) -> Concat_1/9
  Bit_Slice_52/1 -> fa17/2(in2)
  CONST_u1b_0/1 -> Concat_1/32, Concat/1
  fa3/2(C) -> Concat_1/28
  fa17/2(C) -> Concat_1/14
  Bit_Slice_53/1 -> fa17/3(Cin)
  in3/1 -> Bit_Slice_92/1, Bit_Slice_89/1, Bit_Slice_86/1, Bit_Slice_83/1, Bit_Slice_80/1, Bit_Slice_77/1, Bit_Slice_74/1, Bit_Slice_71/1, Bit_Slice_68/1, Bit_Slice_65/1, Bit_Slice_62/1, Bit_Slice_59/1, Bit_Slice_56/1, Bit_Slice_53/1, Bit_Slice_50/1, Bit_Slice_47/1, Bit_Slice_44/1, Bit_Slice_41/1, Bit_Slice_38/1, Bit_Slice_35/1, Bit_Slice_32/1, Bit_Slice_29/1, Bit_Slice_26/1, Bit_Slice_23/1, Bit_Slice_20/1, Bit_Slice_17/1, Bit_Slice_14/1, Bit_Slice_11/1, Bit_Slice_8/1, Bit_Slice_5/1, Bit_Slice_2/1
  fa8/1(S) -> Concat/24
  Bit_Slice_35/1 -> fa11/3(Cin)
  Bit_Slice_51/1 -> fa17/1(in1)
  Bit_Slice_50/1 -> fa16/3(Cin)
  Bit_Slice_30/1 -> fa10/1(in1)
  fa15/2(C) -> Concat_1/16
  fa11/1(S) -> Concat/21
  Bit_Slice_47/1 -> fa15/3(Cin)

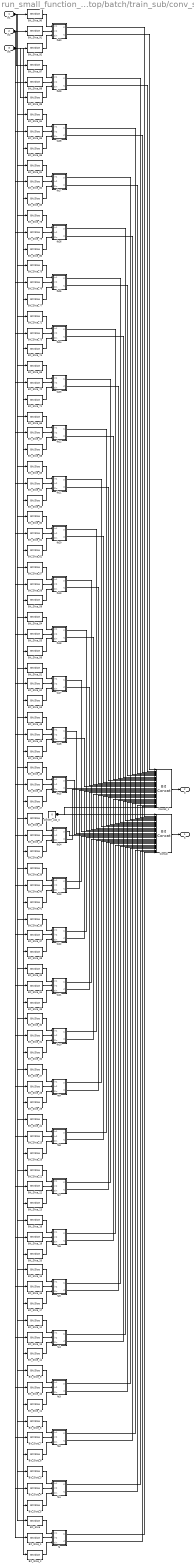
== system run_small_function_cov_bitadder/For Iterator Subsystem/train_top/batch/train_sub/conv_sig/filter dim iter /i ietar Subsystem/Subsystem/For Iterator Subsystem/mac/wt_multi/ca05 ==
  in1 : Inport  OutDataTypeStr=uint32  SampleTime=-1
  in2 : Inport  Port=2  OutDataTypeStr=uint32  SampleTime=-1
  in3 : Inport  Port=3  OutDataTypeStr=uint32  SampleTime=-1
  Bit_Slice : hdlsllib/Logic and Bit Operations/Bit Slice  lidx=double(0)  ridx=double(0)
  Bit_Slice_1 : hdlsllib/Logic and Bit Operations/Bit Slice  lidx=double(0)  ridx=double(0)
  Bit_Slice_10 : hdlsllib/Logic and Bit Operations/Bit Slice  lidx=double(3)  ridx=double(3)
  Bit_Slice_11 : hdlsllib/Logic and Bit Operations/Bit Slice  lidx=double(3)  ridx=double(3)
  Bit_Slice_12 : hdlsllib/Logic and Bit Operations/Bit Slice  lidx=double(4)  ridx=double(4)
  Bit_Slice_13 : hdlsllib/Logic and Bit Operations/Bit Slice  lidx=double(4)  ridx=double(4)
  Bit_Slice_14 : hdlsllib/Logic and Bit Operations/Bit Slice  lidx=double(4)  ridx=double(4)
  Bit_Slice_15 : hdlsllib/Logic and Bit Operations/Bit Slice  lidx=double(5)  ridx=double(5)
  Bit_Slice_16 : hdlsllib/Logic and Bit Operations/Bit Slice  lidx=double(5)  ridx=double(5)
  Bit_Slice_17 : hdlsllib/Logic and Bit Operations/Bit Slice  lidx=double(5)  ridx=double(5)
  Bit_Slice_18 : hdlsllib/Logic and Bit Operations/Bit Slice  lidx=double(6)  ridx=double(6)
  Bit_Slice_19 : hdlsllib/Logic and Bit Operations/Bit Slice  lidx=double(6)  ridx=double(6)
  Bit_Slice_2 : hdlsllib/Logic and Bit Operations/Bit Slice  lidx=double(0)  ridx=double(0)
  Bit_Slice_20 : hdlsllib/Logic and Bit Operations/Bit Slice  lidx=double(6)  ridx=double(6)
  Bit_Slice_21 : hdlsllib/Logic and Bit Operations/Bit Slice  lidx=double(7)  ridx=double(7)
  Bit_Slice_22 : hdlsllib/Logic and Bit Operations/Bit Slice  lidx=double(7)  ridx=double(7)
  Bit_Slice_23 : hdlsllib/Logic and Bit Operations/Bit Slice  lidx=double(7)  ridx=double(7)
  Bit_Slice_24 : hdlsllib/Logic and Bit Operations/Bit Slice  lidx=double(8)  ridx=double(8)
  Bit_Slice_25 : hdlsllib/Logic and Bit Operations/Bit Slice  lidx=double(8)  ridx=double(8)
  Bit_Slice_26 : hdlsllib/Logic and Bit Operations/Bit Slice  lidx=double(8)  ridx=double(8)
  Bit_Slice_27 : hdlsllib/Logic and Bit Operations/Bit Slice  lidx=double(9)  ridx=double(9)
  Bit_Slice_28 : hdlsllib/Logic and Bit Operations/Bit Slice  lidx=double(9)  ridx=double(9)
  Bit_Slice_29 : hdlsllib/Logic and Bit Operations/Bit Slice  lidx=double(9)  ridx=double(9)
  Bit_Slice_3 : hdlsllib/Logic and Bit Operations/Bit Slice  lidx=double(1)  ridx=double(1)
  Bit_Slice_30 : hdlsllib/Logic and Bit Operations/Bit Slice  lidx=double(10)  ridx=double(10)
  Bit_Slice_31 : hdlsllib/Logic and Bit Operations/Bit Slice  lidx=double(10)  ridx=double(10)
  Bit_Slice_32 : hdlsllib/Logic and Bit Operations/Bit Slice  lidx=double(10)  ridx=double(10)
  Bit_Slice_33 : hdlsllib/Logic and Bit Operations/Bit Slice  lidx=double(11)  ridx=double(11)
  Bit_Slice_34 : hdlsllib/Logic and Bit Operations/Bit Slice  lidx=double(11)  ridx=double(11)
  Bit_Slice_35 : hdlsllib/Logic and Bit Operations/Bit Slice  lidx=double(11)  ridx=double(11)
  Bit_Slice_36 : hdlsllib/Logic and Bit Operations/Bit Slice  lidx=double(12)  ridx=double(12)
  Bit_Slice_37 : hdlsllib/Logic and Bit Operations/Bit Slice  lidx=double(12)  ridx=double(12)
  Bit_Slice_38 : hdlsllib/Logic and Bit Operations/Bit Slice  lidx=double(12)  ridx=double(12)
  Bit_Slice_39 : hdlsllib/Logic and Bit Operations/Bit Slice  lidx=double(13)  ridx=double(13)
  Bit_Slice_4 : hdlsllib/Logic and Bit Operations/Bit Slice  lidx=double(1)  ridx=double(1)
  Bit_Slice_40 : hdlsllib/Logic and Bit Operations/Bit Slice  lidx=double(13)  ridx=double(13)
  Bit_Slice_41 : hdlsllib/Logic and Bit Operations/Bit Slice  lidx=double(13)  ridx=double(13)
  Bit_Slice_42 : hdlsllib/Logic and Bit Operations/Bit Slice  lidx=double(14)  ridx=double(14)
  Bit_Slice_43 : hdlsllib/Logic and Bit Operations/Bit Slice  lidx=double(14)  ridx=double(14)
  Bit_Slice_44 : hdlsllib/Logic and Bit Operations/Bit Slice  lidx=double(14)  ridx=double(14)
  Bit_Slice_45 : hdlsllib/Logic and Bit Operations/Bit Slice  lidx=double(15)  ridx=double(15)
  Bit_Slice_46 : hdlsllib/Logic and Bit Operations/Bit Slice  lidx=double(15)  ridx=double(15)
  Bit_Slice_47 : hdlsllib/Logic and Bit Operations/Bit Slice  lidx=double(15)  ridx=double(15)
  Bit_Slice_48 : hdlsllib/Logic and Bit Operations/Bit Slice  lidx=double(16)  ridx=double(16)
  Bit_Slice_49 : hdlsllib/Logic and Bit Operations/Bit Slice  lidx=double(16)  ridx=double(16)
  Bit_Slice_5 : hdlsllib/Logic and Bit Operations/Bit Slice  lidx=double(1)  ridx=double(1)
  Bit_Slice_50 : hdlsllib/Logic and Bit Operations/Bit Slice  lidx=double(16)  ridx=double(16)
  Bit_Slice_51 : hdlsllib/Logic and Bit Operations/Bit Slice  lidx=double(17)  ridx=double(17)
  Bit_Slice_52 : hdlsllib/Logic and Bit Operations/Bit Slice  lidx=double(17)  ridx=double(17)
  Bit_Slice_53 : hdlsllib/Logic and Bit Operations/Bit Slice  lidx=double(17)  ridx=double(17)
  Bit_Slice_54 : hdlsllib/Logic and Bit Operations/Bit Slice  lidx=double(18)  ridx=double(18)
  Bit_Slice_55 : hdlsllib/Logic and Bit Operations/Bit Slice  lidx=double(18)  ridx=double(18)
  Bit_Slice_56 : hdlsllib/Logic and Bit Operations/Bit Slice  lidx=double(18)  ridx=double(18)
  Bit_Slice_57 : hdlsllib/Logic and Bit Operations/Bit Slice  lidx=double(19)  ridx=double(19)
  Bit_Slice_58 : hdlsllib/Logic and Bit Operations/Bit Slice  lidx=double(19)  ridx=double(19)
  Bit_Slice_59 : hdlsllib/Logic and Bit Operations/Bit Slice  lidx=double(19)  ridx=double(19)
  Bit_Slice_6 : hdlsllib/Logic and Bit Operations/Bit Slice  lidx=double(2)  ridx=double(2)
  Bit_Slice_60 : hdlsllib/Logic and Bit Operations/Bit Slice  lidx=double(20)  ridx=double(20)
  Bit_Slice_61 : hdlsllib/Logic and Bit Operations/Bit Slice  lidx=double(20)  ridx=double(20)
  Bit_Slice_62 : hdlsllib/Logic and Bit Operations/Bit Slice  lidx=double(20)  ridx=double(20)
  Bit_Slice_63 : hdlsllib/Logic and Bit Operations/Bit Slice  lidx=double(21)  ridx=double(21)
  Bit_Slice_64 : hdlsllib/Logic and Bit Operations/Bit Slice  lidx=double(21)  ridx=double(21)
  Bit_Slice_65 : hdlsllib/Logic and Bit Operations/Bit Slice  lidx=double(21)  ridx=double(21)
  Bit_Slice_66 : hdlsllib/Logic and Bit Operations/Bit Slice  lidx=double(22)  ridx=double(22)
  Bit_Slice_67 : hdlsllib/Logic and Bit Operations/Bit Slice  lidx=double(22)  ridx=double(22)
  Bit_Slice_68 : hdlsllib/Logic and Bit Operations/Bit Slice  lidx=double(22)  ridx=double(22)
  Bit_Slice_69 : hdlsllib/Logic and Bit Operations/Bit Slice  lidx=double(23)  ridx=double(23)
  Bit_Slice_7 : hdlsllib/Logic and Bit Operations/Bit Slice  lidx=double(2)  ridx=double(2)
  Bit_Slice_70 : hdlsllib/Logic and Bit Operations/Bit Slice  lidx=double(23)  ridx=double(23)
  Bit_Slice_71 : hdlsllib/Logic and Bit Operations/Bit Slice  lidx=double(23)  ridx=double(23)
  Bit_Slice_72 : hdlsllib/Logic and Bit Operations/Bit Slice  lidx=double(24)  ridx=double(24)
  Bit_Slice_73 : hdlsllib/Logic and Bit Operations/Bit Slice  lidx=double(24)  ridx=double(24)
  Bit_Slice_74 : hdlsllib/Logic and Bit Operations/Bit Slice  lidx=double(24)  ridx=double(24)
  Bit_Slice_75 : hdlsllib/Logic and Bit Operations/Bit Slice  lidx=double(25)  ridx=double(25)
  Bit_Slice_76 : hdlsllib/Logic and Bit Operations/Bit Slice  lidx=double(25)  ridx=double(25)
  Bit_Slice_77 : hdlsllib/Logic and Bit Operations/Bit Slice  lidx=double(25)  ridx=double(25)
  Bit_Slice_78 : hdlsllib/Logic and Bit Operations/Bit Slice  lidx=double(26)  ridx=double(26)
  Bit_Slice_79 : hdlsllib/Logic and Bit Operations/Bit Slice  lidx=double(26)  ridx=double(26)
  Bit_Slice_8 : hdlsllib/Logic and Bit Operations/Bit Slice  lidx=double(2)  ridx=double(2)
  Bit_Slice_80 : hdlsllib/Logic and Bit Operations/Bit Slice  lidx=double(26)  ridx=double(26)
  Bit_Slice_81 : hdlsllib/Logic and Bit Operations/Bit Slice  lidx=double(27)  ridx=double(27)
  Bit_Slice_82 : hdlsllib/Logic and Bit Operations/Bit Slice  lidx=double(27)  ridx=double(27)
  Bit_Slice_83 : hdlsllib/Logic and Bit Operations/Bit Slice  lidx=double(27)  ridx=double(27)
  Bit_Slice_84 : hdlsllib/Logic and Bit Operations/Bit Slice  lidx=double(28)  ridx=double(28)
  Bit_Slice_85 : hdlsllib/Logic and Bit Operations/Bit Slice  lidx=double(28)  ridx=double(28)
  Bit_Slice_86 : hdlsllib/Logic and Bit Operations/Bit Slice  lidx=double(28)  ridx=double(28)
  Bit_Slice_87 : hdlsllib/Logic and Bit Operations/Bit Slice  lidx=double(29)  ridx=double(29)
  Bit_Slice_88 : hdlsllib/Logic and Bit Operations/Bit Slice  lidx=double(29)  ridx=double(29)
  Bit_Slice_89 : hdlsllib/Logic and Bit Operations/Bit Slice  lidx=double(29)  ridx=double(29)
  Bit_Slice_9 : hdlsllib/Logic and Bit Operations/Bit Slice  lidx=double(3)  ridx=double(3)
  Bit_Slice_90 : hdlsllib/Logic and Bit Operations/Bit Slice  lidx=double(30)  ridx=double(30)
  Bit_Slice_91 : hdlsllib/Logic and Bit Operations/Bit Slice  lidx=double(30)  ridx=double(30)
  Bit_Slice_92 : hdlsllib/Logic and Bit Operations/Bit Slice  lidx=double(30)  ridx=double(30)
  CONST_u1b_0 : Constant  Value=0  OutDataTypeStr=fixdt(0, 1, 0)  SampleTime=-1
  Concat : hdlsllib/Logic and Bit Operations/Bit Concat  numInputs=32
  Concat_1 : hdlsllib/Logic and Bit Operations/Bit Concat  numInputs=32
  fa : Subsystem
  fa1 : Subsystem
  fa10 : Subsystem
  fa11 : Subsystem
  fa12 : Subsystem
  fa13 : Subsystem
  fa14 : Subsystem
  fa15 : Subsystem
  fa16 : Subsystem
  fa17 : Subsystem
  fa18 : Subsystem
  fa19 : Subsystem
  fa2 : Subsystem
  fa20 : Subsystem
  fa21 : Subsystem
  fa22 : Subsystem
  fa23 : Subsystem
  fa24 : Subsystem
  fa25 : Subsystem
  fa26 : Subsystem
  fa27 : Subsystem
  fa28 : Subsystem
  fa29 : Subsystem
  fa3 : Subsystem
  fa30 : Subsystem
  fa4 : Subsystem
  fa5 : Subsystem
  fa6 : Subsystem
  fa7 : Subsystem
  fa8 : Subsystem
  fa9 : Subsystem
  S : Outport  OutDataTypeStr=uint32  SampleTime=-1
  C : Outport  Port=2  OutDataTypeStr=uint32  SampleTime=-1
  wires:
  in3/1 -> Bit_Slice_92/1, Bit_Slice_89/1, Bit_Slice_86/1, Bit_Slice_83/1, Bit_Slice_80/1, Bit_Slice_77/1, Bit_Slice_74/1, Bit_Slice_71/1, Bit_Slice_68/1, Bit_Slice_65/1, Bit_Slice_62/1, Bit_Slice_59/1, Bit_Slice_56/1, Bit_Slice_53/1, Bit_Slice_50/1, Bit_Slice_47/1, Bit_Slice_44/1, Bit_Slice_41/1, Bit_Slice_38/1, Bit_Slice_35/1, Bit_Slice_32/1, Bit_Slice_29/1, Bit_Slice_26/1, Bit_Slice_23/1, Bit_Slice_20/1, Bit_Slice_17/1, Bit_Slice_14/1, Bit_Slice_11/1, Bit_Slice_8/1, Bit_Slice_5/1, Bit_Slice_2/1
  Concat_1/1 -> C/1
  fa/1(S) -> Concat/32
  fa/2(C) -> Concat_1/31
  Bit_Slice_3/1 -> fa1/1(in1)
  Bit_Slice_5/1 -> fa1/3(Cin)
  fa1/1(S) -> Concat/31
  fa1/2(C) -> Concat_1/30
  Bit_Slice_7/1 -> fa2/2(in2)
  Bit_Slice_9/1 -> fa3/1(in1)
  fa3/1(S) -> Concat/29
  Bit_Slice_12/1 -> fa4/1(in1)
  Bit_Slice_14/1 -> fa4/3(Cin)
  fa4/1(S) -> Concat/28
  Bit_Slice_17/1 -> fa5/3(Cin)
  in2/1 -> Bit_Slice_91/1, Bit_Slice_88/1, Bit_Slice_85/1, Bit_Slice_82/1, Bit_Slice_79/1, Bit_Slice_76/1, Bit_Slice_73/1, Bit_Slice_70/1, Bit_Slice_67/1, Bit_Slice_64/1, Bit_Slice_61/1, Bit_Slice_58/1, Bit_Slice_55/1, Bit_Slice_52/1, Bit_Slice_49/1, Bit_Slice_46/1, Bit_Slice_43/1, Bit_Slice_40/1, Bit_Slice_37/1, Bit_Slice_34/1, Bit_Slice_31/1, Bit_Slice_28/1, Bit_Slice_25/1, Bit_Slice_22/1, Bit_Slice_19/1, Bit_Slice_16/1, Bit_Slice_13/1, Bit_Slice_10/1, Bit_Slice_7/1, Bit_Slice_4/1, Bit_Slice_1/1
  fa5/1(S) -> Concat/27
  fa6/1(S) -> Concat/26
  fa6/2(C) -> Concat_1/25
  Bit_Slice_21/1 -> fa7/1(in1)
  Bit_Slice_22/1 -> fa7/2(in2)
  fa7/1(S) -> Concat/25
  fa7/2(C) -> Concat_1/24
  Bit_Slice_24/1 -> fa8/1(in1)
  Bit_Slice_25/1 -> fa8/2(in2)
  fa8/1(S) -> Concat/24
  fa8/2(C) -> Concat_1/23
  Bit_Slice_28/1 -> fa9/2(in2)
  fa9/1(S) -> Concat/23
  fa9/2(C) -> Concat_1/22
  Bit_Slice_30/1 -> fa10/1(in1)
  Bit_Slice_33/1 -> fa11/1(in1)
  Bit_Slice_36/1 -> fa12/1(in1)
  Bit_Slice_15/1 -> fa5/1(in1)
  Bit_Slice_37/1 -> fa12/2(in2)
  Bit_Slice_26/1 -> fa8/3(Cin)
  fa12/1(S) -> Concat/20
  fa12/2(C) -> Concat_1/19
  Bit_Slice_18/1 -> fa6/1(in1)
  Bit_Slice_39/1 -> fa13/1(in1)
  Bit_Slice_40/1 -> fa13/2(in2)
  Bit_Slice_43/1 -> fa14/2(in2)
  Bit_Slice_34/1 -> fa11/2(in2)
  Bit_Slice_44/1 -> fa14/3(Cin)
  fa14/2(C) -> Concat_1/17
  Bit_Slice_45/1 -> fa15/1(in1)
  Bit_Slice/1 -> fa/1(in1)
  Bit_Slice_19/1 -> fa6/2(in2)
  Bit_Slice_38/1 -> fa12/3(Cin)
  Bit_Slice_46/1 -> fa15/2(in2)
  Bit_Slice_73/1 -> fa24/2(in2)
  in1/1 -> Bit_Slice_90/1, Bit_Slice_87/1, Bit_Slice_84/1, Bit_Slice_81/1, Bit_Slice_78/1, Bit_Slice_75/1, Bit_Slice_72/1, Bit_Slice_69/1, Bit_Slice_66/1, Bit_Slice_63/1, Bit_Slice_60/1, Bit_Slice_57/1, Bit_Slice_54/1, Bit_Slice_51/1, Bit_Slice_48/1, Bit_Slice_45/1, Bit_Slice_42/1, Bit_Slice_39/1, Bit_Slice_36/1, Bit_Slice_33/1, Bit_Slice_30/1, Bit_Slice_27/1, Bit_Slice_24/1, Bit_Slice_21/1, Bit_Slice_18/1, Bit_Slice_15/1, Bit_Slice_12/1, Bit_Slice_9/1, Bit_Slice_6/1, Bit_Slice_3/1, Bit_Slice/1
  Bit_Slice_2/1 -> fa/3(Cin)
  Bit_Slice_74/1 -> fa24/3(Cin)
  fa25/1(S) -> Concat/7
  Bit_Slice_82/1 -> fa27/2(in2)
  fa23/2(C) -> Concat_1/8
  fa25/2(C) -> Concat_1/6
  Concat/1 -> S/1
  fa24/2(C) -> Concat_1/7
  Bit_Slice_92/1 -> fa30/3(Cin)
  fa23/1(S) -> Concat/9
  Bit_Slice_79/1 -> fa26/2(in2)
  fa4/2(C) -> Concat_1/27
  fa26/1(S) -> Concat/6
  fa26/2(C) -> Concat_1/5
  Bit_Slice_76/1 -> fa25/2(in2)
  fa22/2(C) -> Concat_1/9
  fa10/2(C) -> Concat_1/21
  fa27/1(S) -> Concat/5
  Bit_Slice_61/1 -> fa20/2(in2)
  Bit_Slice_72/1 -> fa24/1(in1)
  Bit_Slice_1/1 -> fa/2(in2)
  Bit_Slice_31/1 -> fa10/2(in2)
  fa29/2(C) -> Concat_1/2
  fa2/2(C) -> Concat_1/29
  Bit_Slice_80/1 -> fa26/3(Cin)
  fa29/1(S) -> Concat/3
  Bit_Slice_10/1 -> fa3/2(in2)
  fa5/2(C) -> Concat_1/26
  fa11/1(S) -> Concat/21
  Bit_Slice_86/1 -> fa28/3(Cin)
  Bit_Slice_29/1 -> fa9/3(Cin)
  fa20/1(S) -> Concat/12
  fa30/2(C) -> Concat_1/1
  fa30/1(S) -> Concat/2
  fa28/2(C) -> Concat_1/3
  Bit_Slice_90/1 -> fa30/1(in1)
  fa24/1(S) -> Concat/8
  Bit_Slice_75/1 -> fa25/1(in1)
  Bit_Slice_83/1 -> fa27/3(Cin)
  Bit_Slice_67/1 -> fa22/2(in2)
  Bit_Slice_84/1 -> fa28/1(in1)
  fa28/1(S) -> Concat/4
  Bit_Slice_77/1 -> fa25/3(Cin)
  Bit_Slice_11/1 -> fa3/3(Cin)
  Bit_Slice_85/1 -> fa28/2(in2)
  fa27/2(C) -> Concat_1/4
  Bit_Slice_6/1 -> fa2/1(in1)
  Bit_Slice_51/1 -> fa17/1(in1)
  Bit_Slice_48/1 -> fa16/1(in1)
  Bit_Slice_71/1 -> fa23/3(Cin)
  Bit_Slice_8/1 -> fa2/3(Cin)
  Bit_Slice_32/1 -> fa10/3(Cin)
  Bit_Slice_70/1 -> fa23/2(in2)
  Bit_Slice_35/1 -> fa11/3(Cin)
  Bit_Slice_69/1 -> fa23/1(in1)
  fa2/1(S) -> Concat/30
  fa13/1(S) -> Concat/19
  Bit_Slice_56/1 -> fa18/3(Cin)
  fa14/1(S) -> Concat/18
  Bit_Slice_53/1 -> fa17/3(Cin)
  fa3/2(C) -> Concat_1/28
  Bit_Slice_91/1 -> fa30/2(in2)
  fa22/1(S) -> Concat/10
  Bit_Slice_23/1 -> fa7/3(Cin)
  Bit_Slice_68/1 -> fa22/3(Cin)
  Bit_Slice_81/1 -> fa27/1(in1)
  Bit_Slice_87/1 -> fa29/1(in1)
  Bit_Slice_66/1 -> fa22/1(in1)
  Bit_Slice_65/1 -> fa21/3(Cin)
  Bit_Slice_52/1 -> fa17/2(in2)
  Bit_Slice_64/1 -> fa21/2(in2)
  Bit_Slice_89/1 -> fa29/3(Cin)
  Bit_Slice_63/1 -> fa21/1(in1)
  Bit_Slice_13/1 -> fa4/2(in2)
  Bit_Slice_41/1 -> fa13/3(Cin)
  fa13/2(C) -> Concat_1/18
  fa21/1(S) -> Concat/11
  Bit_Slice_57/1 -> fa19/1(in1)
  Bit_Slice_42/1 -> fa14/1(in1)
  Bit_Slice_78/1 -> fa26/1(in1)
  fa20/2(C) -> Concat_1/11
  Bit_Slice_20/1 -> fa6/3(Cin)
  Bit_Slice_62/1 -> fa20/3(Cin)
  fa21/2(C) -> Concat_1/10
  Bit_Slice_60/1 -> fa20/1(in1)
  fa11/2(C) -> Concat_1/20
  fa19/2(C) -> Concat_1/12
  Bit_Slice_4/1 -> fa1/2(in2)
  Bit_Slice_27/1 -> fa9/1(in1)
  fa19/1(S) -> Concat/13
  CONST_u1b_0/1 -> Concat_1/32, Concat/1
  fa15/1(S) -> Concat/17
  Bit_Slice_59/1 -> fa19/3(Cin)
  Bit_Slice_55/1 -> fa18/2(in2)
  fa17/1(S) -> Concat/15
  Bit_Slice_58/1 -> fa19/2(in2)
  fa18/2(C) -> Concat_1/13
  fa10/1(S) -> Concat/22
  Bit_Slice_88/1 -> fa29/2(in2)
  fa18/1(S) -> Concat/14
  Bit_Slice_54/1 -> fa18/1(in1)
  Bit_Slice_16/1 -> fa5/2(in2)
  Bit_Slice_50/1 -> fa16/3(Cin)
  fa17/2(C) -> Concat_1/14
  fa16/2(C) -> Concat_1/15
  fa16/1(S) -> Concat/16
  Bit_Slice_49/1 -> fa16/2(in2)
  fa15/2(C) -> Concat_1/16
  Bit_Slice_47/1 -> fa15/3(Cin)
